simulink model "SE17"  (R2021a)
settings: Solver=FixedStepAuto  StartTime=0.0  StopTime=20  FixedStep=.01  RelTol=1e-3
undefined symbols (not defined in the file or in its folder): Ion, Li, r_c, r_D, u_ce0, u_D0
libraries: Lib_EMTAT x26, pid_lib x5
(part 1 of 2)
settings Model: PacingRate=0.100000  Creator=mebell  LastModifiedBy=mebell
settings SolverCC: AlgebraicLoopSolver=TrustRegion
settings DebuggingCC: SFMachineParentedDataDiag=warning

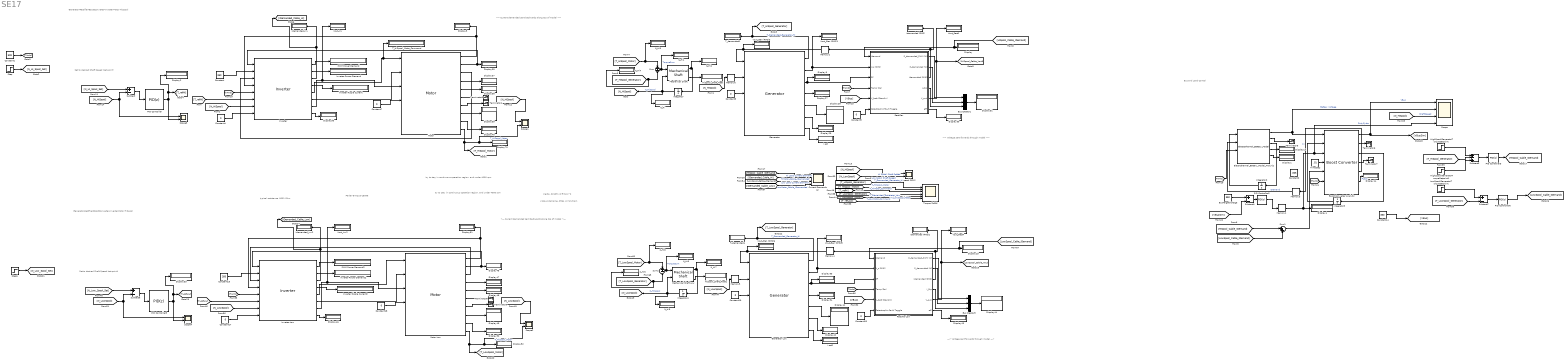
== system SE17 ==
  note: Set to desired Shaft Speed (set point)
  note: Generator-Rectifier-BoostConverter-Inverter-Motor HiSpool
  note: ---> Voltage sent forwards through model --->
  note: <--- Current demanded sent backwards along top of model <---
  note: try to stay in continuous operation region, and under 4000 rpm
  note: Parker GVK210-150N6
  note: typical resistance .0001 Ohm
  note: try to stay in continuous operation region, and under 4000 rpm
  note: viscous damping .2564 x2 Nm/krpm
  note: inertia .02109 x2 ft lbs s^2
  note: Bus and Load Control
  note: Set to desired Shaft Speed (set point)
  note: ---> Voltage sent forwards through model --->
  note: Generator-Rectifier-BoostConverter-Inverter-Motor HiSpool
  note: <--- Current demanded sent backwards along top of model <---
  Boost Converter Analytic : Lib_EMTAT/Components/Physics-Based/Boost Converter  Pdis_M=1  C_M=5e-08  L_M=0.00051  Ron_M=0.784  RC_M=0.26259  RL_M=0.16086  QgTotal_M=4.5e-09  Vdiode_M=0.8  TRise_M=7e-09  TFall_M=2e-09  Fsw_M=250000  Vgate_M=1.7  n_MOSFET=1  MassEst_M=0.37515  TempIn=Celsius  vOut=125  pow=100  minV=47  maxV=53  rippleMode=Use defaults (5% of voltage output and 10% of inductor current)  vRip=.05  iRip=.1  freqMode=Use default frequency (250 kHz)  freq=250e3
      link override DC - DC Converter/Steady State/TemperatureModifiedPerformanceTerm1 /Constant: Value=1
      settings: SourceProductName=EMTAT
  Bus Creator1 : BusCreator  Inputs=3
  Bus Creator3 : BusCreator  Inputs=3
  BusTargetVoltage : Constant  Value=350
  Constant : Constant  Value=350
  Constant1 : Constant  Value=528
  Constant14 : Constant  Value=350
  Constant15 : Constant  Value=350
  Constant{4,7..9,17..20} (8 alike) : Constant  Value=0
  Constant2 : Constant  Value=.005
  Current Demands (A) : Scope  NumInputPorts=4
  Display{,1..2,4..5,9,13..15,27..31,33..53,75} (36 alike) : Display
  Electrothermal_Battery_Model_Analytic : Lib_EMTAT/Components/Physics-Based/Electrothermal_Battery_Model  E0_M=E0_M  Q_M=Q_M  R_M=R_M  K_M=K_M  B_M=B_M  SOC_Init_M=100  A_M=A_M  battery_type_M=Li-Ion  TempIn=Celsius  BWS=on  thermal=on  nameField=Thermal Model
      settings: SourceProductName=EMTAT
  Generator : Lib_EMTAT/Components/Physics-Based/Generator  pp=3  flux_m=0.15995  R_s=0.02  L_s=0.33  P_Fe_Nom=143776.8778  S_nom=4000  T_nom=110  P_out_max=58600  I_max=360.5  P_in_max=81000  T_max=191  MassEst_M=-8670163  Poles_i=6  R_s_i=.02  L_s_i=.330  S_nom_i=4000  T_nom_i=110  P_out_max_i=58600  I_max_i=360.5  P_in_max_i=81000  K_i=50.25  V_nom_i=340  T_max_i=191  CalculatePFe=Compute iron losses automatically  P_Fe_Nom_i=1200  I_nom_i=180  PF_nom_i=0.99  P_Fe_Calc_Flag=1
      settings: SourceProductName=EMTAT
  Generator Low : Lib_EMTAT/Components/Physics-Based/Generator  pp=3  flux_m=0.15995  R_s=0.02  L_s=0.33  P_Fe_Nom=143776.8778  S_nom=4000  T_nom=110  P_out_max=58600  I_max=360.5  P_in_max=81000  T_max=191  MassEst_M=-8670163  Poles_i=6  R_s_i=.02  L_s_i=.330  S_nom_i=4000  T_nom_i=110  P_out_max_i=58600  I_max_i=360.5  P_in_max_i=81000  K_i=50.25  V_nom_i=340  T_max_i=191  CalculatePFe=Compute iron losses automatically  P_Fe_Nom_i=1200  I_nom_i=180  PF_nom_i=0.99  P_Fe_Calc_Flag=1
      settings: SourceProductName=EMTAT
  HiSpool_Shaft_Heat : Display
  HiSpool_Shaft_Heat1 : Display
  HighSpoolGeneratorTorqueSetpoint : Step  Time=7  After=25  SampleTime=0
  HighSpoolGeneratorTorqueSetpoint1 : Step  Time=4  After=-20  SampleTime=0
  I act : Display
  I act2 : Display
  Idemanded (RMS) : Display
  Idemanded (RMS)2 : Display
  Idemanded_inv : Display
  Idemanded_inv2 : Display
  Integrator : Integrator  LimitOutput=on
  Integrator2 : Integrator
  Integrator3 : Integrator
  Integrator4 : Integrator  LimitOutput=on
  "Inverter " : Lib_EMTAT/Components/Physics-Based/Inverter   T_M=[25 175]  u_D_M=[1.16666666666667 0.999999999999998]  u_ce0_M=[0.971428571428571 0.848275862068965]  R_c_M=[0.0285714285714286 0.0551724137931034]  R_D_M=[0.0238095238095238 0.0294117647058824]  E0_M=[6.00000000000002e-05 6.00000000000002e-05]  E1_M=[5.6e-05 5.6e-05]  f_sw_M=20000  L_s_M=0.1  P_max_I=22000  V_phase_I=600  f_sw_I=0  L_s_I=0.1
      settings: SourceProductName=EMTAT
  Inverter Low : Lib_EMTAT/Components/Physics-Based/Inverter   T_M=[25 175]  u_D_M=[1.16666666666667 0.999999999999998]  u_ce0_M=[0.971428571428571 0.848275862068965]  R_c_M=[0.0285714285714286 0.0551724137931034]  R_D_M=[0.0238095238095238 0.0294117647058824]  E0_M=[6.00000000000002e-05 6.00000000000002e-05]  E1_M=[5.6e-05 5.6e-05]  f_sw_M=20000  L_s_M=0.1  P_max_I=22000  V_phase_I=600  f_sw_I=0  L_s_I=0.1
      settings: SourceProductName=EMTAT
  Inverter Power Demand : Display
  Inverter Power Demand2 : Display
  Inverter Ripple Current : Display
  Inverter Ripple Current2 : Display
  LowSpoolGeneratorTorqueSetpoint : Step  Time=12  After=-5  SampleTime=0
  Mechanical Shaft : Lib_EMTAT/Components/Power Flow/Mechanical Shaft  J=.0422  B=.0236
      settings: SourceProductName=EMTAT
      settings: AttributesFormatString=|
      | Mechanical Shaft
      | Version: %<LibraryVersion>
  Mechanical Shaft Low : Lib_EMTAT/Components/Power Flow/Mechanical Shaft  J=.0422  B=.0236
      settings: SourceProductName=EMTAT
      settings: AttributesFormatString=|
      | Mechanical Shaft
      | Version: %<LibraryVersion>
  Memory1 : Memory  InitialCondition=.8
  Memory2 : Memory  InitialCondition=1
  Memory3 : Memory  InitialCondition=.05
  Memory4 : Memory  InitialCondition=1
  Memory5 : Memory  InitialCondition=3000
  Memory6 : Memory  InitialCondition=3000
  "Motor " : Lib_EMTAT/Components/Physics-Based/Motor   pp=6  flux_m=0.079975  R_s=0.02  L_s=0.33  P_Fe_Nom=1200  S_nom=4000  T_nom=110  P_out_max=58600  I_max=360.5  P_in_max=81000  T_max=191  MassEst_M=25  Poles_i=12  R_s_i=.02  L_s_i=.330  S_nom_i=4000  T_nom_i=110  P_out_max_i=58600  I_max_i=360.5  P_in_max_i=81000  K_i=50.25  V_nom_i=340  T_max_i=191  CalculatePFe=Compute iron losses automatically  P_Fe_Nom_i=1200  I_nom_i=180  PF_nom_i=0.99  P_Fe_Calc_Flag=1
      settings: SourceProductName=EMTAT
  Motor Low : Lib_EMTAT/Components/Physics-Based/Motor   pp=6  flux_m=0.079975  R_s=0.02  L_s=0.33  P_Fe_Nom=1200  S_nom=4000  T_nom=110  P_out_max=58600  I_max=360.5  P_in_max=81000  T_max=191  MassEst_M=25  Poles_i=12  R_s_i=.02  L_s_i=.330  S_nom_i=4000  T_nom_i=110  P_out_max_i=58600  I_max_i=360.5  P_in_max_i=81000  K_i=50.25  V_nom_i=340  T_max_i=191  CalculatePFe=Compute iron losses automatically  P_Fe_Nom_i=1200  I_nom_i=180  PF_nom_i=0.99  P_Fe_Calc_Flag=1
      settings: SourceProductName=EMTAT
  N_Hi{,1..9} (10 alike) : Display
  PID Controller : pid_lib/PID Controller  Controller=PID  Form=Parallel  TimeDomain=Discrete-time  UseExternalTs=off  SampleTime=-1  IntegratorMethod=Forward Euler  FilterMethod=Forward Euler  ControllerParametersSource=internal  P=.05  I=.01  D=0  UseFilter=on  N=100  TunerSelectOption=Transfer Function Based (PID Tuner App)  InitialConditionSource=internal  InitialConditionForIntegrator=0  InitialConditionForFilter=0  DifferentiatorICPrevScaledInput=0  ExternalReset=none  TrackingMode=off  Kt=1  LimitOutput=off  SatLimitsSource=internal  UpperSaturationLimit=inf  LowerSaturationLimit=-inf  LinearizeAsGain=on  AntiWindupMode=none  Kb=1  RndMeth=Round  POutMin=[]  POutMax=[]  IOutMin=[]  IOutMax=[]  DOutMin=[]  DOutMax=[]  NOutMin=[]  NOutMax=[]  SumOutMin=[]  SumOutMax=[]  SaturationOutMin=[]  SaturationOutMax=[]  PParamMin=[]  PParamMax=[]  IParamMin=[]  IParamMax=[]  DParamMin=[]  DParamMax=[]  NParamMin=[]  NParamMax=[]  KbParamMin=[]  KbParamMax=[]  KtParamMin=[]  KtParamMax=[]  KbOutMin=[]  KbOutMax=[]  KtOutMin=[]  KtOutMax=[]  IntegratorOutMin=[]  IntegratorOutMax=[]  FilterOutMin=[]  FilterOutMax=[]  SumI1OutMin=[]  SumI1OutMax=[]  SumI2OutMin=[]  SumI2OutMax=[]  SumI3OutMin=[]  SumI3OutMax=[]  SumI4OutMin=[]  SumI4OutMax=[]  SumDOutMin=[]  SumDOutMax=[]  DifferentiatorOutMin=[]  DifferentiatorOutMax=[]  FilterDiffOutCoefMin=[]  FilterDiffOutCoefMax=[]  ReciprocalOutMin=[]  ReciprocalOutMax=[]  SumDenOutMin=[]  SumDenOutMax=[]  SumNumOutMin=[]  SumNumOutMax=[]  DivideOutMin=[]  DivideOutMax=[]  UdiffTsProdOutMin=[]  UdiffTsProdOutMax=[]  NTsProdOutMin=[]  NTsProdOutMax=[]  UintegralTsProdOutMin=[]  UintegralTsProdOutMax=[]  UngainTsProdOutMin=[]  UngainTsProdOutMax=[]  IntegratorContinuousStateAttributes=''  IntegratorStateMustResolveToSignalObject=off  IntegratorRTWStateStorageClass=Auto  FilterContinuousStateAttributes=''  FilterStateMustResolveToSignalObject=off  FilterRTWStateStorageClass=Auto  ParallelPVariant=InternalParameters  IdealPVariant=Disabled  IVariant=InternalParameters  DVariant=InternalParameters  IntegratorVariant=Discrete  SatVariant=Disabled  AWVariant=Passthrough  PCopyVariant=Disabled  TRVariant=Disabled  FdbkBlocksVariant=Forward  IdealPFdbkVariant=Disabled  SatFdbkVariant=Disabled  DerivativeFilterVariant=ForwardEulerFilter  NVariant=InternalParameters  NCopyVariant=Disabled  FilterICVariant=InternalICsFilter  IntegratorICVariant=InternalICs  ExternalResetVariant=Disabled  TRSumVariant=Passthrough  SumFdbkVariant=Disabled  SumVariant=Sum_PID  TsampFilterVariant=InternalTs  TsampNgainVariant=Passthrough  TsampIntegralVariant=Passthrough  ExternalSaturationOutDataTypeStr=Inherit: Same as second input
  PID Controller2 : pid_lib/PID Controller  Controller=PID  Form=Parallel  TimeDomain=Continuous-time  UseExternalTs=off  SampleTime=-1  IntegratorMethod=Forward Euler  FilterMethod=Forward Euler  ControllerParametersSource=internal  P=.0005  I=.005  D=0  UseFilter=on  N=0  TunerSelectOption=Transfer Function Based (PID Tuner App)  InitialConditionSource=internal  InitialConditionForIntegrator=0  InitialConditionForFilter=0  DifferentiatorICPrevScaledInput=0  ExternalReset=none  TrackingMode=off  Kt=1  LimitOutput=on  SatLimitsSource=internal  UpperSaturationLimit=1  LowerSaturationLimit=-inf  LinearizeAsGain=on  AntiWindupMode=none  Kb=1  POutMin=[]  POutMax=[]  IOutMin=[]  IOutMax=[]  DOutMin=[]  DOutMax=[]  NOutMin=[]  NOutMax=[]  SumOutMin=[]  SumOutMax=[]  SaturationOutMin=[]  SaturationOutMax=[]  PParamMin=[]  PParamMax=[]  IParamMin=[]  IParamMax=[]  DParamMin=[]  DParamMax=[]  NParamMin=[]  NParamMax=[]  KbParamMin=[]  KbParamMax=[]  KtParamMin=[]  KtParamMax=[]  KbOutMin=[]  KbOutMax=[]  KtOutMin=[]  KtOutMax=[]  IntegratorOutMin=[]  IntegratorOutMax=[]  FilterOutMin=[]  FilterOutMax=[]  SumI1OutMin=[]  SumI1OutMax=[]  SumI2OutMin=[]  SumI2OutMax=[]  SumI3OutMin=[]  SumI3OutMax=[]  SumI4OutMin=[]  SumI4OutMax=[]  SumDOutMin=[]  SumDOutMax=[]  DifferentiatorOutMin=[]  DifferentiatorOutMax=[]  FilterDiffOutCoefMin=[]  FilterDiffOutCoefMax=[]  ReciprocalOutMin=[]  ReciprocalOutMax=[]  SumDenOutMin=[]  SumDenOutMax=[]  SumNumOutMin=[]  SumNumOutMax=[]  DivideOutMin=[]  DivideOutMax=[]  UdiffTsProdOutMin=[]  UdiffTsProdOutMax=[]  NTsProdOutMin=[]  NTsProdOutMax=[]  UintegralTsProdOutMin=[]  UintegralTsProdOutMax=[]  UngainTsProdOutMin=[]  UngainTsProdOutMax=[]  IntegratorContinuousStateAttributes=''  IntegratorStateMustResolveToSignalObject=off  IntegratorRTWStateStorageClass=Auto  FilterContinuousStateAttributes=''  FilterStateMustResolveToSignalObject=off  FilterRTWStateStorageClass=Auto  ParallelPVariant=InternalParameters  IdealPVariant=Disabled  IVariant=InternalParameters  DVariant=InternalParameters  IntegratorVariant=Continuous  SatVariant=Enabled  AWVariant=Passthrough  PCopyVariant=Disabled  TRVariant=Disabled  FdbkBlocksVariant=Forward  IdealPFdbkVariant=Disabled  SatFdbkVariant=Disabled  DerivativeFilterVariant=ContFilter  NVariant=InternalParameters  NCopyVariant=Disabled  FilterICVariant=InternalICsFilter  IntegratorICVariant=InternalICs  ExternalResetVariant=Disabled  TRSumVariant=Passthrough  SumFdbkVariant=Disabled  SumVariant=Sum_PID  TsampFilterVariant=InternalTs  TsampNgainVariant=Passthrough  TsampIntegralVariant=Passthrough  ExternalSaturationOutDataTypeStr=Inherit: Same as second input
  PID Controller3 : pid_lib/PID Controller  Controller=PID  Form=Parallel  TimeDomain=Continuous-time  UseExternalTs=off  SampleTime=-1  IntegratorMethod=Forward Euler  FilterMethod=Forward Euler  ControllerParametersSource=internal  P=0  I=1.09  D=0  UseFilter=on  N=100  TunerSelectOption=Transfer Function Based (PID Tuner App)  ZeroCross=off  InitialConditionSource=internal  InitialConditionForIntegrator=0  InitialConditionForFilter=0  DifferentiatorICPrevScaledInput=0  ExternalReset=none  TrackingMode=off  Kt=1  LimitOutput=off  SatLimitsSource=internal  UpperSaturationLimit=inf  LowerSaturationLimit=-inf  LinearizeAsGain=on  AntiWindupMode=none  Kb=1  POutMin=[]  POutMax=[]  IOutMin=[]  IOutMax=[]  DOutMin=[]  DOutMax=[]  NOutMin=[]  NOutMax=[]  SumOutMin=[]  SumOutMax=[]  SaturationOutMin=[]  SaturationOutMax=[]  PParamMin=[]  PParamMax=[]  IParamMin=[]  IParamMax=[]  DParamMin=[]  DParamMax=[]  NParamMin=[]  NParamMax=[]  KbParamMin=[]  KbParamMax=[]  KtParamMin=[]  KtParamMax=[]  KbOutMin=[]  KbOutMax=[]  KtOutMin=[]  KtOutMax=[]  IntegratorOutMin=[]  IntegratorOutMax=[]  FilterOutMin=[]  FilterOutMax=[]  SumI1OutMin=[]  SumI1OutMax=[]  SumI2OutMin=[]  SumI2OutMax=[]  SumI3OutMin=[]  SumI3OutMax=[]  SumI4OutMin=[]  SumI4OutMax=[]  SumDOutMin=[]  SumDOutMax=[]  DifferentiatorOutMin=[]  DifferentiatorOutMax=[]  FilterDiffOutCoefMin=[]  FilterDiffOutCoefMax=[]  ReciprocalOutMin=[]  ReciprocalOutMax=[]  SumDenOutMin=[]  SumDenOutMax=[]  SumNumOutMin=[]  SumNumOutMax=[]  DivideOutMin=[]  DivideOutMax=[]  UdiffTsProdOutMin=[]  UdiffTsProdOutMax=[]  NTsProdOutMin=[]  NTsProdOutMax=[]  UintegralTsProdOutMin=[]  UintegralTsProdOutMax=[]  UngainTsProdOutMin=[]  UngainTsProdOutMax=[]  IntegratorContinuousStateAttributes=''  IntegratorStateMustResolveToSignalObject=off  IntegratorRTWStateStorageClass=Auto  FilterContinuousStateAttributes=''  FilterStateMustResolveToSignalObject=off  FilterRTWStateStorageClass=Auto  ParallelPVariant=InternalParameters  IdealPVariant=Disabled  IVariant=InternalParameters  DVariant=InternalParameters  IntegratorVariant=Continuous  SatVariant=Disabled  AWVariant=Passthrough  PCopyVariant=Disabled  TRVariant=Disabled  FdbkBlocksVariant=Forward  IdealPFdbkVariant=Disabled  SatFdbkVariant=Disabled  DerivativeFilterVariant=ContFilter  NVariant=InternalParameters  NCopyVariant=Disabled  FilterICVariant=InternalICsFilter  IntegratorICVariant=InternalICs  ExternalResetVariant=Disabled  TRSumVariant=Passthrough  SumFdbkVariant=Disabled  SumVariant=Sum_PID  TsampFilterVariant=InternalTs  TsampNgainVariant=Passthrough  TsampIntegralVariant=Passthrough  ExternalSaturationOutDataTypeStr=Inherit: Same as second input
  PID Controller5 : pid_lib/PID Controller  Controller=PID  Form=Parallel  TimeDomain=Discrete-time  UseExternalTs=off  SampleTime=-1  IntegratorMethod=Forward Euler  FilterMethod=Forward Euler  ControllerParametersSource=internal  P=.05  I=.01  D=0  UseFilter=on  N=100  TunerSelectOption=Transfer Function Based (PID Tuner App)  InitialConditionSource=internal  InitialConditionForIntegrator=0  InitialConditionForFilter=0  DifferentiatorICPrevScaledInput=0  ExternalReset=none  TrackingMode=off  Kt=1  LimitOutput=off  SatLimitsSource=internal  UpperSaturationLimit=inf  LowerSaturationLimit=-inf  LinearizeAsGain=on  AntiWindupMode=none  Kb=1  RndMeth=Round  POutMin=[]  POutMax=[]  IOutMin=[]  IOutMax=[]  DOutMin=[]  DOutMax=[]  NOutMin=[]  NOutMax=[]  SumOutMin=[]  SumOutMax=[]  SaturationOutMin=[]  SaturationOutMax=[]  PParamMin=[]  PParamMax=[]  IParamMin=[]  IParamMax=[]  DParamMin=[]  DParamMax=[]  NParamMin=[]  NParamMax=[]  KbParamMin=[]  KbParamMax=[]  KtParamMin=[]  KtParamMax=[]  KbOutMin=[]  KbOutMax=[]  KtOutMin=[]  KtOutMax=[]  IntegratorOutMin=[]  IntegratorOutMax=[]  FilterOutMin=[]  FilterOutMax=[]  SumI1OutMin=[]  SumI1OutMax=[]  SumI2OutMin=[]  SumI2OutMax=[]  SumI3OutMin=[]  SumI3OutMax=[]  SumI4OutMin=[]  SumI4OutMax=[]  SumDOutMin=[]  SumDOutMax=[]  DifferentiatorOutMin=[]  DifferentiatorOutMax=[]  FilterDiffOutCoefMin=[]  FilterDiffOutCoefMax=[]  ReciprocalOutMin=[]  ReciprocalOutMax=[]  SumDenOutMin=[]  SumDenOutMax=[]  SumNumOutMin=[]  SumNumOutMax=[]  DivideOutMin=[]  DivideOutMax=[]  UdiffTsProdOutMin=[]  UdiffTsProdOutMax=[]  NTsProdOutMin=[]  NTsProdOutMax=[]  UintegralTsProdOutMin=[]  UintegralTsProdOutMax=[]  UngainTsProdOutMin=[]  UngainTsProdOutMax=[]  IntegratorContinuousStateAttributes=''  IntegratorStateMustResolveToSignalObject=off  IntegratorRTWStateStorageClass=Auto  FilterContinuousStateAttributes=''  FilterStateMustResolveToSignalObject=off  FilterRTWStateStorageClass=Auto  ParallelPVariant=InternalParameters  IdealPVariant=Disabled  IVariant=InternalParameters  DVariant=InternalParameters  IntegratorVariant=Discrete  SatVariant=Disabled  AWVariant=Passthrough  PCopyVariant=Disabled  TRVariant=Disabled  FdbkBlocksVariant=Forward  IdealPFdbkVariant=Disabled  SatFdbkVariant=Disabled  DerivativeFilterVariant=ForwardEulerFilter  NVariant=InternalParameters  NCopyVariant=Disabled  FilterICVariant=InternalICsFilter  IntegratorICVariant=InternalICs  ExternalResetVariant=Disabled  TRSumVariant=Passthrough  SumFdbkVariant=Disabled  SumVariant=Sum_PID  TsampFilterVariant=InternalTs  TsampNgainVariant=Passthrough  TsampIntegralVariant=Passthrough  ExternalSaturationOutDataTypeStr=Inherit: Same as second input
  PID Controller6 : pid_lib/PID Controller  Controller=PID  Form=Parallel  TimeDomain=Continuous-time  UseExternalTs=off  SampleTime=-1  IntegratorMethod=Forward Euler  FilterMethod=Forward Euler  ControllerParametersSource=internal  P=0  I=1.09  D=0  UseFilter=on  N=100  TunerSelectOption=Transfer Function Based (PID Tuner App)  ZeroCross=off  InitialConditionSource=internal  InitialConditionForIntegrator=0  InitialConditionForFilter=0  DifferentiatorICPrevScaledInput=0  ExternalReset=none  TrackingMode=off  Kt=1  LimitOutput=off  SatLimitsSource=internal  UpperSaturationLimit=inf  LowerSaturationLimit=-inf  LinearizeAsGain=on  AntiWindupMode=none  Kb=1  POutMin=[]  POutMax=[]  IOutMin=[]  IOutMax=[]  DOutMin=[]  DOutMax=[]  NOutMin=[]  NOutMax=[]  SumOutMin=[]  SumOutMax=[]  SaturationOutMin=[]  SaturationOutMax=[]  PParamMin=[]  PParamMax=[]  IParamMin=[]  IParamMax=[]  DParamMin=[]  DParamMax=[]  NParamMin=[]  NParamMax=[]  KbParamMin=[]  KbParamMax=[]  KtParamMin=[]  KtParamMax=[]  KbOutMin=[]  KbOutMax=[]  KtOutMin=[]  KtOutMax=[]  IntegratorOutMin=[]  IntegratorOutMax=[]  FilterOutMin=[]  FilterOutMax=[]  SumI1OutMin=[]  SumI1OutMax=[]  SumI2OutMin=[]  SumI2OutMax=[]  SumI3OutMin=[]  SumI3OutMax=[]  SumI4OutMin=[]  SumI4OutMax=[]  SumDOutMin=[]  SumDOutMax=[]  DifferentiatorOutMin=[]  DifferentiatorOutMax=[]  FilterDiffOutCoefMin=[]  FilterDiffOutCoefMax=[]  ReciprocalOutMin=[]  ReciprocalOutMax=[]  SumDenOutMin=[]  SumDenOutMax=[]  SumNumOutMin=[]  SumNumOutMax=[]  DivideOutMin=[]  DivideOutMax=[]  UdiffTsProdOutMin=[]  UdiffTsProdOutMax=[]  NTsProdOutMin=[]  NTsProdOutMax=[]  UintegralTsProdOutMin=[]  UintegralTsProdOutMax=[]  UngainTsProdOutMin=[]  UngainTsProdOutMax=[]  IntegratorContinuousStateAttributes=''  IntegratorStateMustResolveToSignalObject=off  IntegratorRTWStateStorageClass=Auto  FilterContinuousStateAttributes=''  FilterStateMustResolveToSignalObject=off  FilterRTWStateStorageClass=Auto  ParallelPVariant=InternalParameters  IdealPVariant=Disabled  IVariant=InternalParameters  DVariant=InternalParameters  IntegratorVariant=Continuous  SatVariant=Disabled  AWVariant=Passthrough  PCopyVariant=Disabled  TRVariant=Disabled  FdbkBlocksVariant=Forward  IdealPFdbkVariant=Disabled  SatFdbkVariant=Disabled  DerivativeFilterVariant=ContFilter  NVariant=InternalParameters  NCopyVariant=Disabled  FilterICVariant=InternalICsFilter  IntegratorICVariant=InternalICs  ExternalResetVariant=Disabled  TRSumVariant=Passthrough  SumFdbkVariant=Disabled  SumVariant=Sum_PID  TsampFilterVariant=InternalTs  TsampNgainVariant=Passthrough  TsampIntegralVariant=Passthrough  ExternalSaturationOutDataTypeStr=Inherit: Same as second input
  PWM Power Demand : Display
  PWM Power Demand2 : Display
  Rectifier : Subsystem  AncestorBlock=Lib_EMTAT/Components/Physics-Based/Rectifier  mask{T_M=[25 175], u_D_M=[1.16666666666667 0.999999999999998], u_ce0_M=[0.971428571428571 0.848275862068965], R_c_M=[0.0285714285714286 0.0551724137931034], R_D_M=[0.0238095238095238 0.0294117647058824], E0_M=[6.00000000000002e-05 6.00000000000002e-05], E1_M=[5.6e-05 5.6e-05], f_sw_M=20000, L_s_M=0.1, P_max_I=22000, V_phase_I=600, f_sw_I=0, L_s_I=0.1}
      mask prompts: T_M "Temperature Breakpoints (degrees C)"; u_D_M "u_D (Diode voltage at 0A), as a function of T"; u_ce0_M "u_ce0 (IGBT voltage at 0A), as a function of T"; R_c_M "R_c (IGBT resistance), as a function of T"; R_D_M "R_D (Diode resistance), as a linear of T"; E0_M "E0 switching energy coefficient"; E1_M "E1 switching energy coefficient"; f_sw_M "Switching Frequency (Hz)"; L_s_M "Stator Inductance of Attached Motor"; P_max_I "Maximum power"; V_phase_I "Maximum phase voltage (set to 0 to disregard)"; f_sw_I "F_sw (set to 0 to default to maximum for given IGBT)"; L_s_I "Stator inductance of Motor (required for ripple current calculation)"
      mask DialogControl Container4 Prompt: Parameters
      mask DialogControl Control2 Prompt: The way that the above parameters are used is that each vector is 2 long, using points in the linear zone of the curves. Interpolation is used to find values at other temperatures.
      mask DialogControl Container4_copy Prompt: iDesign 1
      mask DialogControl runbutton Prompt: RUN iDESIGN
      mask DialogControl runbutton Callback: run('Run_iDesign_InverterSS')
  Rectifier Low : Subsystem  AncestorBlock=Lib_EMTAT/Components/Physics-Based/Rectifier  mask{T_M=[25 175], u_D_M=[1.16666666666667 0.999999999999998], u_ce0_M=[0.971428571428571 0.848275862068965], R_c_M=[0.0285714285714286 0.0551724137931034], R_D_M=[0.0238095238095238 0.0294117647058824], E0_M=[6.00000000000002e-05 6.00000000000002e-05], E1_M=[5.6e-05 5.6e-05], f_sw_M=20000, L_s_M=0.1, P_max_I=22000, V_phase_I=600, f_sw_I=0, L_s_I=0.1}
      mask prompts: T_M "Temperature Breakpoints (degrees C)"; u_D_M "u_D (Diode voltage at 0A), as a function of T"; u_ce0_M "u_ce0 (IGBT voltage at 0A), as a function of T"; R_c_M "R_c (IGBT resistance), as a function of T"; R_D_M "R_D (Diode resistance), as a linear of T"; E0_M "E0 switching energy coefficient"; E1_M "E1 switching energy coefficient"; f_sw_M "Switching Frequency (Hz)"; L_s_M "Stator Inductance of Attached Motor"; P_max_I "Maximum power"; V_phase_I "Maximum phase voltage (set to 0 to disregard)"; f_sw_I "F_sw (set to 0 to default to maximum for given IGBT)"; L_s_I "Stator inductance of Motor (required for ripple current calculation)"
      mask DialogControl Container4 Prompt: Parameters
      mask DialogControl Control2 Prompt: The way that the above parameters are used is that each vector is 2 long, using points in the linear zone of the curves. Interpolation is used to find values at other temperatures.
      mask DialogControl Container4_copy Prompt: iDesign 1
      mask DialogControl runbutton Prompt: RUN iDESIGN
      mask DialogControl runbutton Callback: run('Run_iDesign_InverterSS')
  Scope : Scope  NumInputPorts=4
  Scope{1..4} (4 alike) : Scope  NumInputPorts=2
  Speed (RPM) : Scope  NumInputPorts=2
  Step : Step  Time=.5  After=4000  SampleTime=0
  Step6 : Step  Time=.75  After=4000  SampleTime=0
  Subtract{,1,6..7} (4 alike) : Sum  Inputs=+-
  Subtract3 : Sum  Inputs=+-+
  Sum : Sum  Inputs=+|-
  Sum1 : Sum  Inputs=|++
  Sum2 : Sum  Inputs=+|-
  T_HiSpool_Motor_Command : Display
  T_demanded1 : Display
  T_demanded4 : Display
  Terminator{3..9} (7 alike) : Terminator
  TimeStep : Constant  Value=.01
  Torque (lbf-ft) : Scope  NumInputPorts=6
  Vout_Gen (RMS){1,3,5..6} (4 alike) : Display
  Vout_Inv : Display
  Vout_Inv2 : Display
  Vout_Rect1 : Display
  Vout_Rect4 : Display
  wires:
  "Inverter "/6 -> "Motor "/2
  Generator/4 -> Display27/1
  "Motor "/3 -> "Inverter "/3
  Constant1/1 -> [TAmb]
  "Inverter "/7 -> "Motor "/3, Vout_Inv/1
  "Motor "/2 -> "Inverter "/1, Display35/1
  "Motor "/10 -> Scope1/2, Display75/1, [T_HiSpool_Motor]  "T_HiSpool_Motor"
  "Motor "/8 -> Display39/1
  Rectifier/1(P_demanded_PWM (W)) -> Bus Creator1/1
  Generator/7 -> I act/1
  [T_refHi] -> "Inverter "/6
  [TAmb] -> "Inverter "/5
  Rectifier/4(I_Rip) -> Bus Creator1/3
  Bus Creator1/1 -> Display31/1
  Generator/5 -> Display28/1
  Rectifier/5(V_out) -> [HiSpool_Cable_Vout], Vout_Rect1/1
  Generator/3 -> Rectifier/3(PF), Display9/1
  [TAmb] -> Rectifier/4(Temp (Ra))
  Rectifier/6(eff) -> Display30/1
  "Motor "/5 -> Display38/1
  "Motor "/4 -> Display37/1
  "Motor "/9 -> Display40/1
  Generator/6 -> Display29/1
  [N_HiSpool] -> "Inverter "/7
  [N_HiSpool] -> Memory6/1
  "Inverter "/3 -> [IDemanded_Cable_Hi], Idemanded_inv/1
  "Inverter "/8 -> Display36/1
  Rectifier/2(P_demanded (W)) -> Bus Creator1/2
  Rectifier/3(Idemanded (RMS)) -> Idemanded (RMS)/1, Memory2/1
  "Inverter "/5 -> T_HiSpool_Motor_Command/1, "Motor "/1
  Generator/1 -> [T_HiSpool_Generator], T_demanded1/1  "T_Demanded_Generator_Hi"
  Sum/1 -> N_Hi1/1, Mechanical Shaft/1  "TorqueSum"
  Constant/1 -> "Inverter "/2
  [T_HiSpool_Motor] -> N_Hi3/1, Sum/1
  [T_HiSpool_Generator] -> N_Hi4/1, Sum/2
  Mechanical Shaft/3 -> HiSpool_Shaft_Heat/1
  [N_Hi_Spool_Set] -> Subtract/1
  [HiSpool_Cable_IDemand] -> Rectifier/1(Idemand), Display/1
  "Motor "/1 -> "Inverter "/4, Display5/1
  Mechanical Shaft/1 -> N_Hi2/1, Integrator/1
  Integrator/1 -> N_Hi/1, Mechanical Shaft/2, [N_HiSpool]  "N_HiSpool"
  [N_HiSpool] -> Scope1/1
  Generator/2 -> Rectifier/2("V_s (RMS) "), Vout_Gen (RMS)1/1
  [N_HiSpool] -> Speed (RPM)/1  "Hi Spool Shaft Speed"
  PID Controller/1 -> Scope3/2, Display2/1, [T_refHi]
  [N_HiSpool] -> Scope3/1, Subtract/2
  Subtract/1 -> PID Controller/1
  "Inverter "/1 -> PWM Power Demand/1
  "Inverter "/2 -> Inverter Power Demand/1
  Memory6/1 -> Generator/2
  [T_refHi] -> Torque (lbf-ft)/3  "T_HiMotor_Command"
  [HiSpool_Cable_IDemand] -> Current Demands (A)/1  "Hi Load Current Demand"
  [T_HiSpool_Generator] -> Torque (lbf-ft)/1  "T_Demanded_Generator_Hi"
  "Inverter "/4 -> Inverter Ripple Current/1
  "Motor "/7 -> Terminator4/1
  "Motor "/6 -> Terminator3/1
  [TAmb] -> Electrothermal_Battery_Model_Analytic/3
  Electrothermal_Battery_Model_Analytic/1 -> Boost Converter Analytic/1, Scope/2  "Battery Voltage"
  Electrothermal_Battery_Model_Analytic/3 -> Integrator2/1
  Integrator2/1 -> Electrothermal_Battery_Model_Analytic/1
  Electrothermal_Battery_Model_Analytic/2 -> Terminator5/1
  Boost Converter Analytic/5 -> Memory3/1  "Iin"
  Boost Converter Analytic/6 -> Display14/1  "PLoss"
  Electrothermal_Battery_Model_Analytic/4 -> Display13/1
  Boost Converter Analytic/3 -> Integrator3/1
  Integrator3/1 -> Boost Converter Analytic/2
  Boost Converter Analytic/2 -> Terminator6/1
  Boost Converter Analytic/1 -> [VBusSim], Scope/1  "VBus"
  [VBus] -> Rectifier/5(V_batt (Standin))
  Subtract1/1 -> PID Controller2/1
  BusTargetVoltage/1 -> Subtract1/1
  [VBusSim] -> Subtract1/2
  PID Controller2/1 -> Memory1/1
  TimeStep/1 -> Boost Converter Analytic/4
  [TAmb] -> Boost Converter Analytic/6
  Boost Converter Analytic/4 -> Terminator7/1
  Sum1/1 -> Boost Converter Analytic/5
  [N_HiSpool] -> Scope/3  "ShaftSpeed"
  Memory3/1 -> Electrothermal_Battery_Model_Analytic/2  "IDemand"
  Memory1/1 -> Display4/1, Scope/4, Boost Converter Analytic/3  "DutyCycle"
  Step/1 -> [N_Hi_Spool_Set]
  [IDemanded_Cable_Hi] -> Current Demands (A)/2  "HiMotor_Cable_IDemanded"
  Constant4/1 -> "Inverter "/8
  Constant7/1 -> "Motor "/4
  Constant8/1 -> Generator/3
  Constant9/1 -> Rectifier/6(Catastrophic Fault Toggle)
  Memory2/1 -> Vout_Gen (RMS)3/1, Generator/1
  PID Controller3/1 -> [HiSpool_Cable_IDemand]
  Subtract3/1 -> PID Controller3/1
  [T_HiSpool_Generator] -> Subtract3/2
  HighSpoolGeneratorTorqueSetpoint/1 -> Subtract3/1
  Constant14/1 -> [VBus]
  [T_LowSpool_Motor] -> Torque (lbf-ft)/5  "T_LowSpool_Motor"
  [T_HiSpool_Motor] -> Torque (lbf-ft)/2  "T_HiSpool_Motor"
  Mechanical Shaft Low/1 -> N_Hi7/1, Integrator4/1
  Motor Low/5 -> Display48/1
  [LowSpool_Cable_IDemand] -> Rectifier Low/1(Idemand), Display15/1
  Rectifier Low/1(P_demanded_PWM (W)) -> Bus Creator3/1
  Rectifier Low/2(P_demanded (W)) -> Bus Creator3/2
  [TAmb] -> Rectifier Low/4(Temp (Ra))
  Memory4/1 -> Vout_Gen (RMS)6/1, Generator Low/1
  Mechanical Shaft Low/3 -> HiSpool_Shaft_Heat1/1
  Generator Low/2 -> Rectifier Low/2("V_s (RMS) "), Vout_Gen (RMS)5/1
  [N_LowSpool] -> Scope2/1
  Motor Low/1 -> Inverter Low/4, Display51/1
  [N_LowSpool] -> Speed (RPM)/2  "Low Spool Shaft Speed"
  [LowSpool_Cable_IDemand] -> Current Demands (A)/3  "Low Load Current Demand"
  Inverter Low/2 -> Inverter Power Demand2/1
  Generator Low/7 -> I act2/1
  Memory5/1 -> Generator Low/2
  Rectifier Low/3(Idemanded (RMS)) -> Idemanded (RMS)2/1, Memory4/1
  [N_Low_Spool_Set] -> Subtract6/1
  Constant15/1 -> Inverter Low/2
  Inverter Low/1 -> PWM Power Demand2/1
  Subtract6/1 -> PID Controller5/1
  [T_LowSpool_Generator] -> N_Hi9/1, Sum2/2
  Generator Low/1 -> [T_LowSpool_Generator], T_demanded4/1  "T_Demanded_Generator_Hi"
  Inverter Low/3 -> [IDemanded_Cable_Low], Idemanded_inv2/1
  Inverter Low/8 -> Display46/1
  [N_LowSpool] -> Memory5/1
  Generator Low/5 -> Display41/1
  Motor Low/10 -> Scope2/2, Display52/1, [T_LowSpool_Motor]  "T_HiSpool_Motor"
  Motor Low/8 -> Display49/1
  Generator Low/4 -> Display34/1
  Integrator4/1 -> N_Hi5/1, Mechanical Shaft Low/2, [N_LowSpool]  "N_HiSpool"
  Generator Low/3 -> Rectifier Low/3(PF), Display53/1
  Motor Low/9 -> Display50/1
  Constant18/1 -> Motor Low/4
  Constant17/1 -> Inverter Low/8
  [IDemanded_Cable_Low] -> Current Demands (A)/4  "LowMotor_Cable_IDemanded"
  Bus Creator3/1 -> Display44/1
  [T_LowSpool_Generator] -> Torque (lbf-ft)/4  "T_Demanded_Generator_Low"
  [N_LowSpool] -> Scope4/1, Subtract6/2
  Constant20/1 -> Rectifier Low/6(Catastrophic Fault Toggle)
  Step6/1 -> [N_Low_Spool_Set]
  [T_refLow] -> Inverter Low/6
  Rectifier Low/6(eff) -> Display43/1
  Constant19/1 -> Generator Low/3
  PID Controller5/1 -> Scope4/2, Display33/1, [T_refLow]
  Motor Low/3 -> Inverter Low/3
  [VBus] -> Rectifier Low/5(V_batt (Standin))
  Rectifier Low/4(I_Rip) -> Bus Creator3/3
  Inverter Low/7 -> Motor Low/3, Vout_Inv2/1
  Inverter Low/4 -> Inverter Ripple Current2/1
  [N_LowSpool] -> Inverter Low/7
  [T_LowSpool_Motor] -> N_Hi8/1, Sum2/1
  Motor Low/6 -> Terminator8/1
  Inverter Low/5 -> Motor Low/1
  Motor Low/2 -> Inverter Low/1, Display45/1
  Rectifier Low/5(V_out) -> [LowSpool_Cable_Vout], Vout_Rect4/1
  Motor Low/7 -> Terminator9/1
  Generator Low/6 -> Display42/1
  Motor Low/4 -> Display47/1
  [T_refLow] -> Torque (lbf-ft)/6  "T_LowMotor_Command"
  [TAmb] -> Inverter Low/5
  Inverter Low/6 -> Motor Low/2
  Sum2/1 -> N_Hi6/1, Mechanical Shaft Low/1  "TorqueSum"
  [T_LowSpool_Generator] -> Subtract7/2
  PID Controller6/1 -> [LowSpool_Cable_IDemand]
  Subtract7/1 -> PID Controller6/1
  LowSpoolGeneratorTorqueSetpoint/1 -> Subtract7/1
  HighSpoolGeneratorTorqueSetpoint1/1 -> Subtract3/3
  [HiSpool_Cable_IDemand] -> Sum1/1
  [LowSpool_Cable_IDemand] -> Sum1/2
  Electrothermal_Battery_Model_Analytic/5 -> Display1/1

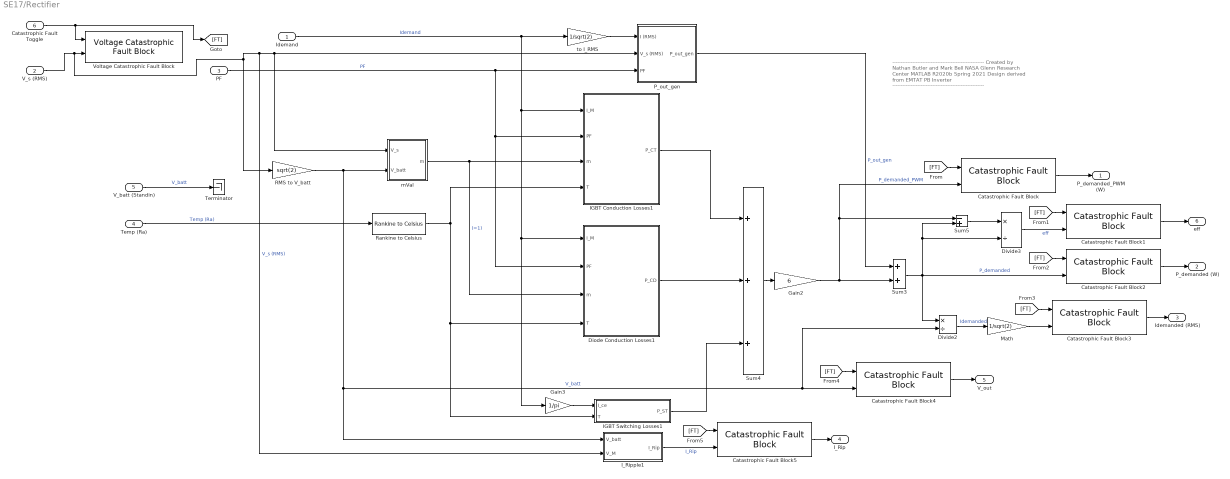
== system SE17/Rectifier ==
  note: -------------------------------------------------------
      | Created by Nathan Butler and Mark Bell
      | NASA Glenn Research Center
      | MATLAB R2020b
      | Spring 2021
      |
      | Design derived from EMTAT PB Inverter
      | -------------------------------------------------------
  Idemand : Inport
  "V_s (RMS) " : Inport  Port=2
  PF : Inport  Port=3
  Temp (Ra) : Inport  Port=4
  V_batt (Standin) : Inport  Port=5
  Catastrophic Fault Toggle : Inport  Port=6
  Catastrophic Fault Block{,1..5} (6 alike) : Lib_EMTAT/Components/Physics-Based/Catastrophic Fault Block  SystemSampleTime=-1  VariantActivationTime=update diagram  Latency=0  AutoFrameSizeCalculation=off
      settings: SourceProductName=EMTAT
  Diode Conduction Losses1 : Subsystem
  Divide2 : Product  Inputs=*/
  Divide3 : Product  Inputs=*/
  Gain2 : Gain  Gain=6
  Gain3 : Gain  Gain=1/pi
  IGBT Conduction Losses1 : Subsystem
  IGBT Switching Losses1 : Subsystem
  I_Ripple1 : Subsystem
  Math : Gain  Gain=1/sqrt(2)
  P_out_gen : Subsystem
  "RMS to V_batt " : Gain  Gain=sqrt(2)
  Rankine to Celsius : Lib_EMTAT/Components/Physics-Based/Rankine to Celsius  SystemSampleTime=-1  VariantActivationTime=update diagram  Latency=0  AutoFrameSizeCalculation=off
      settings: SourceProductName=EMTAT
  Sum3 : Sum
  Sum4 : Sum  Inputs=+++
  Sum5 : Sum  Inputs=-+
  Terminator : Terminator
  Voltage Catastrophic Fault Block : Lib_EMTAT/Components/Physics-Based/Voltage Catastrophic Fault Block  SystemSampleTime=-1  VariantActivationTime=update diagram  Latency=0  AutoFrameSizeCalculation=off
      settings: SourceProductName=EMTAT
  mVal : Subsystem
  to I_RMS : Gain  Gain=1/sqrt(2)
  P_demanded_PWM (W) : Outport  VectorParamsAs1DForOutWhenUnconnected=off
  P_demanded (W) : Outport  Port=2  VectorParamsAs1DForOutWhenUnconnected=off
  Idemanded (RMS) : Outport  Port=3  VectorParamsAs1DForOutWhenUnconnected=off
  I_Rip : Outport  Port=4  VectorParamsAs1DForOutWhenUnconnected=off
  V_out : Outport  Port=5  VectorParamsAs1DForOutWhenUnconnected=off
  eff : Outport  Port=6  VectorParamsAs1DForOutWhenUnconnected=off
  wires:
  "V_s (RMS) "/1 -> P_out_gen/2(V_s (RMS)), mVal/1(V_s), I_Ripple1/2("V_M "), "RMS to V_batt "/1, Voltage Catastrophic Fault Block/2  "V_s (RMS)"
  Catastrophic Fault Toggle/1 -> [FT], Voltage Catastrophic Fault Block/1
  Catastrophic Fault Block5/1 -> I_Rip/1
  I_Ripple1/1(I_Rip) -> Catastrophic Fault Block5/2  "I_Rip"
  [FT] -> Catastrophic Fault Block5/1
  Catastrophic Fault Block4/1 -> V_out/1
  [FT] -> Catastrophic Fault Block4/1
  Catastrophic Fault Block3/1 -> Idemanded (RMS)/1
  Math/1 -> Catastrophic Fault Block3/2
  [FT] -> Catastrophic Fault Block3/1
  Catastrophic Fault Block2/1 -> P_demanded (W)/1
  [FT] -> Catastrophic Fault Block2/1
  Catastrophic Fault Block1/1 -> eff/1
  Divide3/1 -> Catastrophic Fault Block1/2  "eff"
  [FT] -> Catastrophic Fault Block1/1
  [FT] -> Catastrophic Fault Block/1
  Catastrophic Fault Block/1 -> P_demanded_PWM (W)/1
  V_batt (Standin)/1 -> Terminator/1  "V_batt"
  to I_RMS/1 -> P_out_gen/1(I (RMS))
  Sum5/1 -> Divide3/1
  Sum3/1 -> Divide2/1, Sum5/2, Divide3/2, Catastrophic Fault Block2/2  "P_demanded"
  Temp (Ra)/1 -> Rankine to Celsius/1  "Temp (Ra)"
  Gain3/1 -> IGBT Switching Losses1/1(I_ce)
  IGBT Switching Losses1/1(P_ST) -> Sum4/3
  IGBT Conduction Losses1/1(P_CT) -> Sum4/1
  Sum4/1 -> Gain2/1
  Diode Conduction Losses1/1(P_CD) -> Sum4/2
  mVal/1(m) -> IGBT Conduction Losses1/3(m), Diode Conduction Losses1/3(m)  "(=1)"
  PF/1 -> IGBT Conduction Losses1/2(PF), Diode Conduction Losses1/2(PF), P_out_gen/3(PF)  "PF"
  Idemand/1 -> to I_RMS/1, Diode Conduction Losses1/1(I_M), Gain3/1, IGBT Conduction Losses1/1(I_M)  "Idemand"
  Gain2/1 -> Sum5/1, Catastrophic Fault Block/2, Sum3/2  "P_demanded_PWM"
  P_out_gen/1(P_out_gen) -> Sum3/1  "P_out_gen"
  Divide2/1 -> Math/1  "Idemanded"
  "RMS to V_batt "/1 -> mVal/2(V_batt), I_Ripple1/1(V_batt), Divide2/2, Catastrophic Fault Block4/2  "V_batt"
  Rankine to Celsius/1 -> Diode Conduction Losses1/4(T), IGBT Switching Losses1/2(T), IGBT Conduction Losses1/4(T)

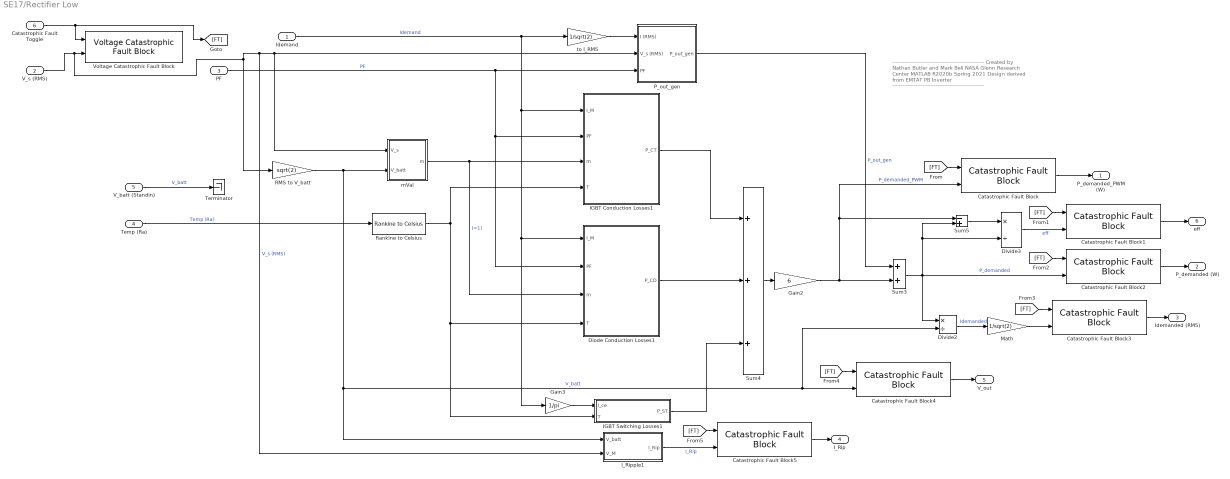
== system SE17/Rectifier Low ==
  note: -------------------------------------------------------
      | Created by Nathan Butler and Mark Bell
      | NASA Glenn Research Center
      | MATLAB R2020b
      | Spring 2021
      |
      | Design derived from EMTAT PB Inverter
      | -------------------------------------------------------
  Idemand : Inport
  "V_s (RMS) " : Inport  Port=2
  PF : Inport  Port=3
  Temp (Ra) : Inport  Port=4
  V_batt (Standin) : Inport  Port=5
  Catastrophic Fault Toggle : Inport  Port=6
  Catastrophic Fault Block{,1..5} (6 alike) : Lib_EMTAT/Components/Physics-Based/Catastrophic Fault Block  SystemSampleTime=-1  VariantActivationTime=update diagram  Latency=0  AutoFrameSizeCalculation=off
      settings: SourceProductName=EMTAT
  Diode Conduction Losses1 : Subsystem
  Divide2 : Product  Inputs=*/
  Divide3 : Product  Inputs=*/
  Gain2 : Gain  Gain=6
  Gain3 : Gain  Gain=1/pi
  IGBT Conduction Losses1 : Subsystem
  IGBT Switching Losses1 : Subsystem
  I_Ripple1 : Subsystem
  Math : Gain  Gain=1/sqrt(2)
  P_out_gen : Subsystem
  "RMS to V_batt " : Gain  Gain=sqrt(2)
  Rankine to Celsius : Lib_EMTAT/Components/Physics-Based/Rankine to Celsius  SystemSampleTime=-1  VariantActivationTime=update diagram  Latency=0  AutoFrameSizeCalculation=off
      settings: SourceProductName=EMTAT
  Sum3 : Sum
  Sum4 : Sum  Inputs=+++
  Sum5 : Sum  Inputs=-+
  Terminator : Terminator
  Voltage Catastrophic Fault Block : Lib_EMTAT/Components/Physics-Based/Voltage Catastrophic Fault Block  SystemSampleTime=-1  VariantActivationTime=update diagram  Latency=0  AutoFrameSizeCalculation=off
      settings: SourceProductName=EMTAT
  mVal : Subsystem
  to I_RMS : Gain  Gain=1/sqrt(2)
  P_demanded_PWM (W) : Outport  VectorParamsAs1DForOutWhenUnconnected=off
  P_demanded (W) : Outport  Port=2  VectorParamsAs1DForOutWhenUnconnected=off
  Idemanded (RMS) : Outport  Port=3  VectorParamsAs1DForOutWhenUnconnected=off
  I_Rip : Outport  Port=4  VectorParamsAs1DForOutWhenUnconnected=off
  V_out : Outport  Port=5  VectorParamsAs1DForOutWhenUnconnected=off
  eff : Outport  Port=6  VectorParamsAs1DForOutWhenUnconnected=off
  wires:
  "V_s (RMS) "/1 -> P_out_gen/2(V_s (RMS)), mVal/1(V_s), I_Ripple1/2("V_M "), "RMS to V_batt "/1, Voltage Catastrophic Fault Block/2  "V_s (RMS)"
  Catastrophic Fault Toggle/1 -> [FT], Voltage Catastrophic Fault Block/1
  Catastrophic Fault Block5/1 -> I_Rip/1
  I_Ripple1/1(I_Rip) -> Catastrophic Fault Block5/2  "I_Rip"
  [FT] -> Catastrophic Fault Block5/1
  Catastrophic Fault Block4/1 -> V_out/1
  [FT] -> Catastrophic Fault Block4/1
  Catastrophic Fault Block3/1 -> Idemanded (RMS)/1
  Math/1 -> Catastrophic Fault Block3/2
  [FT] -> Catastrophic Fault Block3/1
  Catastrophic Fault Block2/1 -> P_demanded (W)/1
  [FT] -> Catastrophic Fault Block2/1
  Catastrophic Fault Block1/1 -> eff/1
  Divide3/1 -> Catastrophic Fault Block1/2  "eff"
  [FT] -> Catastrophic Fault Block1/1
  [FT] -> Catastrophic Fault Block/1
  Catastrophic Fault Block/1 -> P_demanded_PWM (W)/1
  V_batt (Standin)/1 -> Terminator/1  "V_batt"
  to I_RMS/1 -> P_out_gen/1(I (RMS))
  Sum5/1 -> Divide3/1
  Sum3/1 -> Divide2/1, Sum5/2, Divide3/2, Catastrophic Fault Block2/2  "P_demanded"
  Temp (Ra)/1 -> Rankine to Celsius/1  "Temp (Ra)"
  Gain3/1 -> IGBT Switching Losses1/1(I_ce)
  IGBT Switching Losses1/1(P_ST) -> Sum4/3
  IGBT Conduction Losses1/1(P_CT) -> Sum4/1
  Sum4/1 -> Gain2/1
  Diode Conduction Losses1/1(P_CD) -> Sum4/2
  mVal/1(m) -> IGBT Conduction Losses1/3(m), Diode Conduction Losses1/3(m)  "(=1)"
  PF/1 -> IGBT Conduction Losses1/2(PF), Diode Conduction Losses1/2(PF), P_out_gen/3(PF)  "PF"
  Idemand/1 -> to I_RMS/1, Diode Conduction Losses1/1(I_M), Gain3/1, IGBT Conduction Losses1/1(I_M)  "Idemand"
  Gain2/1 -> Sum5/1, Catastrophic Fault Block/2, Sum3/2  "P_demanded_PWM"
  P_out_gen/1(P_out_gen) -> Sum3/1  "P_out_gen"
  Divide2/1 -> Math/1  "Idemanded"
  "RMS to V_batt "/1 -> mVal/2(V_batt), I_Ripple1/1(V_batt), Divide2/2, Catastrophic Fault Block4/2  "V_batt"
  Rankine to Celsius/1 -> Diode Conduction Losses1/4(T), IGBT Switching Losses1/2(T), IGBT Conduction Losses1/4(T)

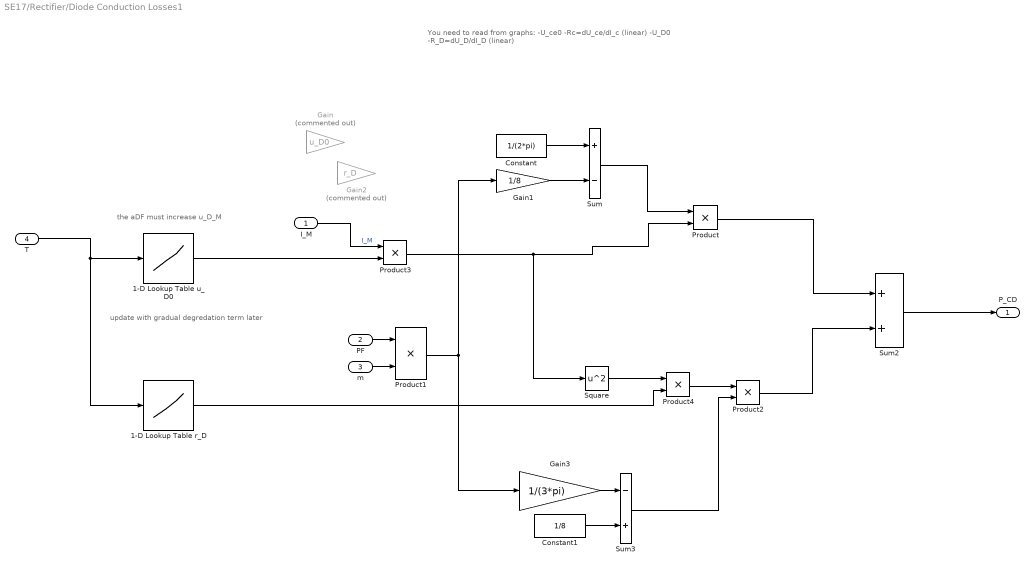
== system SE17/Rectifier/Diode Conduction Losses1 ==
  note: You need to read from graphs:
      |
      | -U_ce0
      | -Rc=dU_ce/dI_c (linear)
      | -U_D0
      | -R_D=dU_D/dI_D (linear)
  note: the aDF must increase u_D_M
  note: update with gradual degredation term later
  I_M : Inport
  PF : Inport  Port=2
  m : Inport  Port=3
  T : Inport  Port=4
  1-D Lookup Table r_D : Lookup_n-D  NumberOfTableDimensions=1  BreakpointsForDimension1=T_M  Table=R_D_M  InternalRulePriority=Speed  RndMeth=Simplest  InputSameDT=on
  1-D Lookup Table u_D0 : Lookup_n-D  NumberOfTableDimensions=1  BreakpointsForDimension1=T_M  Table=u_D_M  InternalRulePriority=Speed  RndMeth=Simplest  InputSameDT=on
  Constant : Constant  Value=1/(2*pi)
  Constant1 : Constant  Value=1/8
  Gain : Gain  Commented=on  Gain=u_D0
  Gain1 : Gain  Gain=1/8
  Gain2 : Gain  Commented=on  Gain=r_D
  Gain3 : Gain  Gain=1/(3*pi)
  Product{,1..4} (5 alike) : Product
  Square : Math  Operator=square  SignedPower=on  SaturateOnIntegerOverflow=on
  Sum : Sum  Inputs=+-
  Sum2 : Sum
  Sum3 : Sum  Inputs=-+
  P_CD : Outport  VectorParamsAs1DForOutWhenUnconnected=off
  wires:
  Product/1 -> Sum2/1
  Product2/1 -> Sum2/2
  Sum2/1 -> P_CD/1
  I_M/1 -> Product3/1  "I_M"
  Product3/1 -> Product/2, Square/1
  Constant/1 -> Sum/1
  PF/1 -> Product1/1
  m/1 -> Product1/2
  Gain1/1 -> Sum/2
  Product1/1 -> Gain3/1, Gain1/1
  Sum/1 -> Product/1
  Square/1 -> Product4/1
  Gain3/1 -> Sum3/1
  Product4/1 -> Product2/1
  Constant1/1 -> Sum3/2
  Sum3/1 -> Product2/2
  T/1 -> 1-D Lookup Table u_D0/1, 1-D Lookup Table r_D/1
  1-D Lookup Table u_D0/1 -> Product3/2
  1-D Lookup Table r_D/1 -> Product4/2

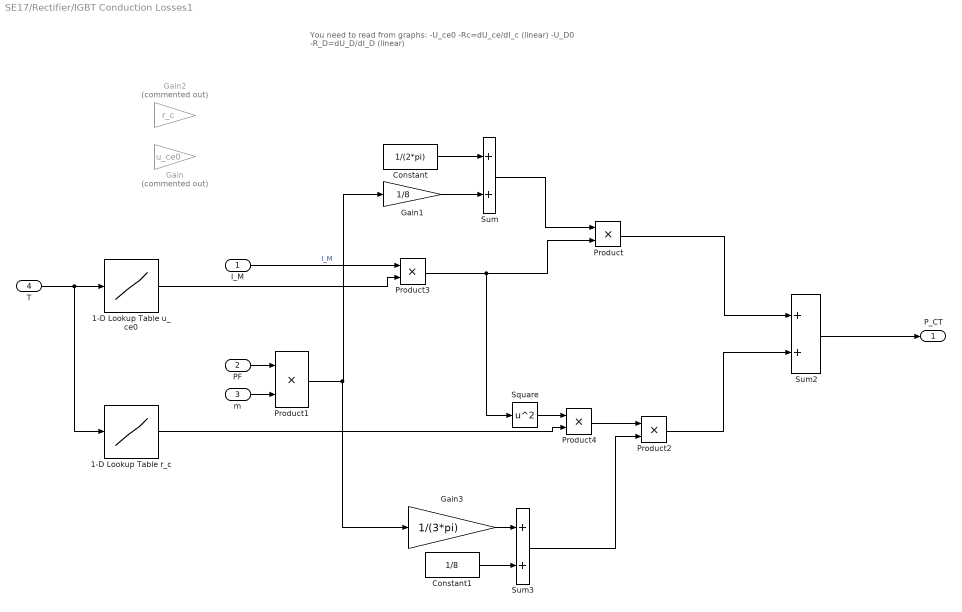
== system SE17/Rectifier/IGBT Conduction Losses1 ==
  note: You need to read from graphs:
      |
      | -U_ce0
      | -Rc=dU_ce/dI_c (linear)
      | -U_D0
      | -R_D=dU_D/dI_D (linear)
  I_M : Inport
  PF : Inport  Port=2
  m : Inport  Port=3
  T : Inport  Port=4
  1-D Lookup Table r_c : Lookup_n-D  NumberOfTableDimensions=1  BreakpointsForDimension1=T_M  Table=R_c_M  InternalRulePriority=Speed  RndMeth=Simplest  InputSameDT=on
  1-D Lookup Table u_ce0 : Lookup_n-D  NumberOfTableDimensions=1  BreakpointsForDimension1=T_M  Table=u_ce0_M  InternalRulePriority=Speed  RndMeth=Simplest  InputSameDT=on
  Constant : Constant  Value=1/(2*pi)
  Constant1 : Constant  Value=1/8
  Gain : Gain  Commented=on  Gain=u_ce0
  Gain1 : Gain  Gain=1/8
  Gain2 : Gain  Commented=on  Gain=r_c
  Gain3 : Gain  Gain=1/(3*pi)
  Product{,1..4} (5 alike) : Product
  Square : Math  Operator=square  SignedPower=on  SaturateOnIntegerOverflow=on
  Sum : Sum
  Sum2 : Sum
  Sum3 : Sum
  P_CT : Outport  VectorParamsAs1DForOutWhenUnconnected=off
  wires:
  Product/1 -> Sum2/1
  Product2/1 -> Sum2/2
  Sum2/1 -> P_CT/1
  I_M/1 -> Product3/1  "I_M"
  Product3/1 -> Product/2, Square/1
  Constant/1 -> Sum/1
  PF/1 -> Product1/1
  m/1 -> Product1/2
  Gain1/1 -> Sum/2
  Product1/1 -> Gain3/1, Gain1/1
  Sum/1 -> Product/1
  Square/1 -> Product4/1
  Gain3/1 -> Sum3/1
  Product4/1 -> Product2/1
  Constant1/1 -> Sum3/2
  Sum3/1 -> Product2/2
  T/1 -> 1-D Lookup Table u_ce0/1, 1-D Lookup Table r_c/1
  1-D Lookup Table u_ce0/1 -> Product3/2
  1-D Lookup Table r_c/1 -> Product4/2

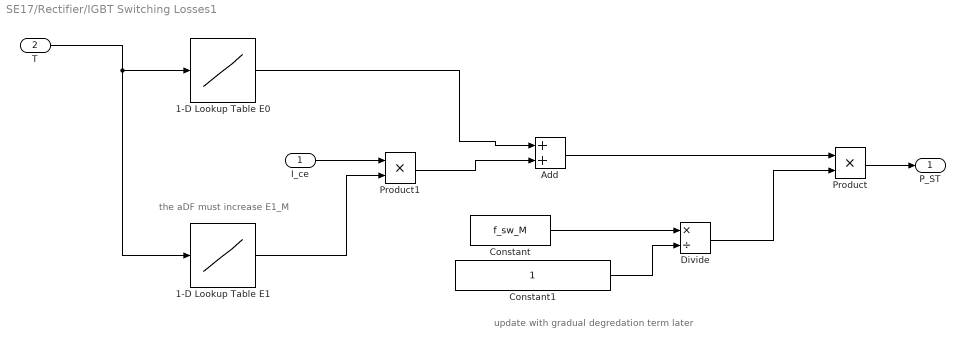
== system SE17/Rectifier/IGBT Switching Losses1 ==
  note: update with gradual degredation term later
  note: the aDF must increase E1_M
  I_ce : Inport
  T : Inport  Port=2
  1-D Lookup Table E0 : Lookup_n-D  NumberOfTableDimensions=1  BreakpointsForDimension1=T_M  Table=E0_M  InternalRulePriority=Speed  RndMeth=Simplest  InputSameDT=on
  1-D Lookup Table E1 : Lookup_n-D  NumberOfTableDimensions=1  BreakpointsForDimension1=T_M  Table=E1_M  InternalRulePriority=Speed  RndMeth=Simplest  InputSameDT=on
  Add : Sum
  Constant : Constant  Value=f_sw_M
  Constant1 : Constant
  Divide : Product  Inputs=*/
  Product : Product
  Product1 : Product
  P_ST : Outport  VectorParamsAs1DForOutWhenUnconnected=off
  wires:
  Constant1/1 -> Divide/2
  Divide/1 -> Product/2
  Constant/1 -> Divide/1
  1-D Lookup Table E1/1 -> Product1/2
  T/1 -> 1-D Lookup Table E1/1, 1-D Lookup Table E0/1
  Product1/1 -> Add/2
  1-D Lookup Table E0/1 -> Add/1
  I_ce/1 -> Product1/1
  Add/1 -> Product/1
  Product/1 -> P_ST/1

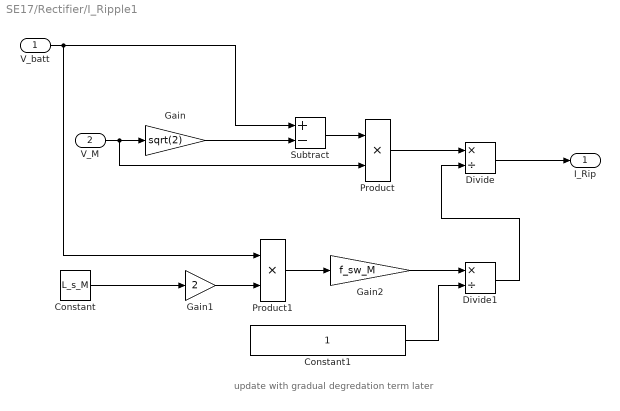
== system SE17/Rectifier/I_Ripple1 ==
  note: update with gradual degredation term later
  V_batt : Inport
  "V_M " : Inport  Port=2
  Constant : Constant  Value=L_s_M
  Constant1 : Constant
  Divide : Product  Inputs=*/
  Divide1 : Product  Inputs=*/
  Gain : Gain  Gain=sqrt(2)
  Gain1 : Gain  Gain=2
  Gain2 : Gain  Gain=f_sw_M
  Product : Product
  Product1 : Product
  Subtract : Sum  Inputs=+-
  I_Rip : Outport  VectorParamsAs1DForOutWhenUnconnected=off
  wires:
  Divide1/1 -> Divide/2
  Constant1/1 -> Divide1/2
  Gain2/1 -> Divide1/1
  "V_M "/1 -> Product/2, Gain/1
  Gain/1 -> Subtract/2
  V_batt/1 -> Subtract/1, Product1/1
  Subtract/1 -> Product/1
  Product/1 -> Divide/1
  Constant/1 -> Gain1/1
  Gain1/1 -> Product1/2
  Product1/1 -> Gain2/1
  Divide/1 -> I_Rip/1

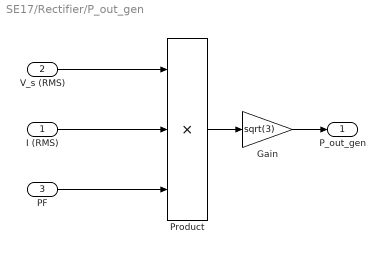
== system SE17/Rectifier/P_out_gen ==
  I (RMS) : Inport
  V_s (RMS) : Inport  Port=2
  PF : Inport  Port=3
  Gain : Gain  Gain=sqrt(3)
  Product : Product  Inputs=3
  P_out_gen : Outport  VectorParamsAs1DForOutWhenUnconnected=off
  wires:
  I (RMS)/1 -> Product/2
  PF/1 -> Product/3
  V_s (RMS)/1 -> Product/1
  Gain/1 -> P_out_gen/1
  Product/1 -> Gain/1

== system SE17/Rectifier/mVal ==
  V_s : Inport
  V_batt : Inport  Port=2
  Divide : Product  Inputs=*/
  Gain : Gain  Gain=sqrt(2)
  m : Outport  VectorParamsAs1DForOutWhenUnconnected=off
  wires:
  Divide/1 -> m/1
  V_s/1 -> Gain/1
  Gain/1 -> Divide/1
  V_batt/1 -> Divide/2

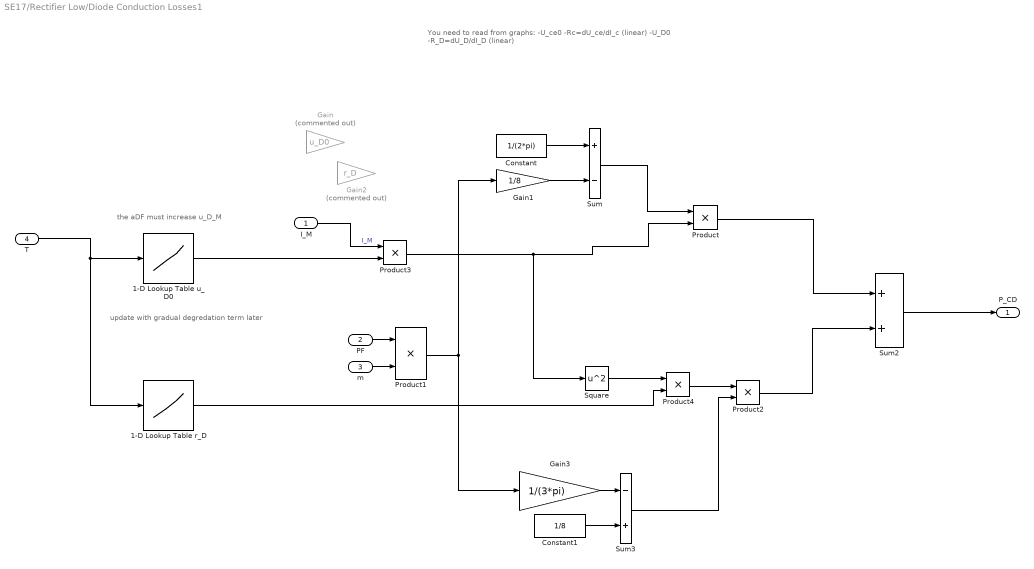
== system SE17/Rectifier Low/Diode Conduction Losses1 ==
  note: You need to read from graphs:
      |
      | -U_ce0
      | -Rc=dU_ce/dI_c (linear)
      | -U_D0
      | -R_D=dU_D/dI_D (linear)
  note: the aDF must increase u_D_M
  note: update with gradual degredation term later
  I_M : Inport
  PF : Inport  Port=2
  m : Inport  Port=3
  T : Inport  Port=4
  1-D Lookup Table r_D : Lookup_n-D  NumberOfTableDimensions=1  BreakpointsForDimension1=T_M  Table=R_D_M  InternalRulePriority=Speed  RndMeth=Simplest  InputSameDT=on
  1-D Lookup Table u_D0 : Lookup_n-D  NumberOfTableDimensions=1  BreakpointsForDimension1=T_M  Table=u_D_M  InternalRulePriority=Speed  RndMeth=Simplest  InputSameDT=on
  Constant : Constant  Value=1/(2*pi)
  Constant1 : Constant  Value=1/8
  Gain : Gain  Commented=on  Gain=u_D0
  Gain1 : Gain  Gain=1/8
  Gain2 : Gain  Commented=on  Gain=r_D
  Gain3 : Gain  Gain=1/(3*pi)
  Product{,1..4} (5 alike) : Product
  Square : Math  Operator=square  SignedPower=on  SaturateOnIntegerOverflow=on
  Sum : Sum  Inputs=+-
  Sum2 : Sum
  Sum3 : Sum  Inputs=-+
  P_CD : Outport  VectorParamsAs1DForOutWhenUnconnected=off
  wires:
  Product/1 -> Sum2/1
  Product2/1 -> Sum2/2
  Sum2/1 -> P_CD/1
  I_M/1 -> Product3/1  "I_M"
  Product3/1 -> Product/2, Square/1
  Constant/1 -> Sum/1
  PF/1 -> Product1/1
  m/1 -> Product1/2
  Gain1/1 -> Sum/2
  Product1/1 -> Gain3/1, Gain1/1
  Sum/1 -> Product/1
  Square/1 -> Product4/1
  Gain3/1 -> Sum3/1
  Product4/1 -> Product2/1
  Constant1/1 -> Sum3/2
  Sum3/1 -> Product2/2
  T/1 -> 1-D Lookup Table u_D0/1, 1-D Lookup Table r_D/1
  1-D Lookup Table u_D0/1 -> Product3/2
  1-D Lookup Table r_D/1 -> Product4/2

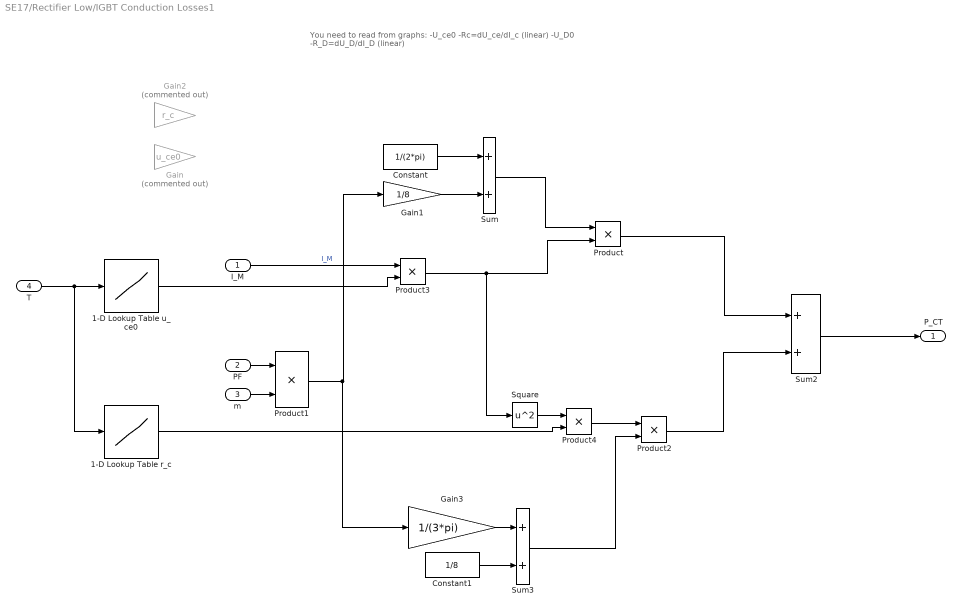
== system SE17/Rectifier Low/IGBT Conduction Losses1 ==
  note: You need to read from graphs:
      |
      | -U_ce0
      | -Rc=dU_ce/dI_c (linear)
      | -U_D0
      | -R_D=dU_D/dI_D (linear)
  I_M : Inport
  PF : Inport  Port=2
  m : Inport  Port=3
  T : Inport  Port=4
  1-D Lookup Table r_c : Lookup_n-D  NumberOfTableDimensions=1  BreakpointsForDimension1=T_M  Table=R_c_M  InternalRulePriority=Speed  RndMeth=Simplest  InputSameDT=on
  1-D Lookup Table u_ce0 : Lookup_n-D  NumberOfTableDimensions=1  BreakpointsForDimension1=T_M  Table=u_ce0_M  InternalRulePriority=Speed  RndMeth=Simplest  InputSameDT=on
  Constant : Constant  Value=1/(2*pi)
  Constant1 : Constant  Value=1/8
  Gain : Gain  Commented=on  Gain=u_ce0
  Gain1 : Gain  Gain=1/8
  Gain2 : Gain  Commented=on  Gain=r_c
  Gain3 : Gain  Gain=1/(3*pi)
  Product{,1..4} (5 alike) : Product
  Square : Math  Operator=square  SignedPower=on  SaturateOnIntegerOverflow=on
  Sum : Sum
  Sum2 : Sum
  Sum3 : Sum
  P_CT : Outport  VectorParamsAs1DForOutWhenUnconnected=off
  wires:
  Product/1 -> Sum2/1
  Product2/1 -> Sum2/2
  Sum2/1 -> P_CT/1
  I_M/1 -> Product3/1  "I_M"
  Product3/1 -> Product/2, Square/1
  Constant/1 -> Sum/1
  PF/1 -> Product1/1
  m/1 -> Product1/2
  Gain1/1 -> Sum/2
  Product1/1 -> Gain3/1, Gain1/1
  Sum/1 -> Product/1
  Square/1 -> Product4/1
  Gain3/1 -> Sum3/1
  Product4/1 -> Product2/1
  Constant1/1 -> Sum3/2
  Sum3/1 -> Product2/2
  T/1 -> 1-D Lookup Table u_ce0/1, 1-D Lookup Table r_c/1
  1-D Lookup Table u_ce0/1 -> Product3/2
  1-D Lookup Table r_c/1 -> Product4/2

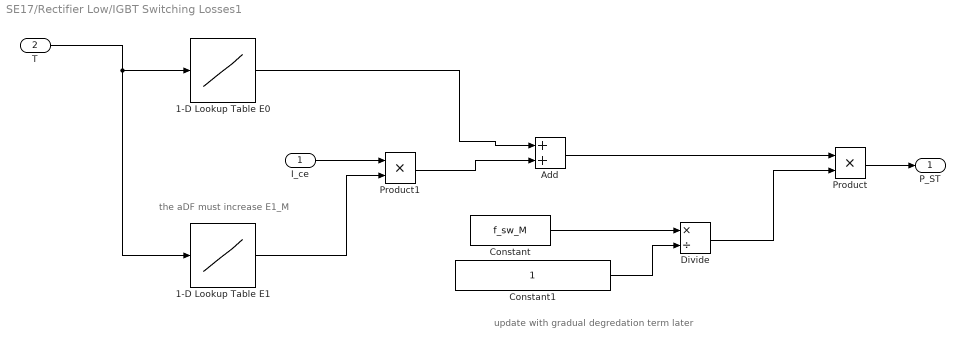
== system SE17/Rectifier Low/IGBT Switching Losses1 ==
  note: update with gradual degredation term later
  note: the aDF must increase E1_M
  I_ce : Inport
  T : Inport  Port=2
  1-D Lookup Table E0 : Lookup_n-D  NumberOfTableDimensions=1  BreakpointsForDimension1=T_M  Table=E0_M  InternalRulePriority=Speed  RndMeth=Simplest  InputSameDT=on
  1-D Lookup Table E1 : Lookup_n-D  NumberOfTableDimensions=1  BreakpointsForDimension1=T_M  Table=E1_M  InternalRulePriority=Speed  RndMeth=Simplest  InputSameDT=on
  Add : Sum
  Constant : Constant  Value=f_sw_M
  Constant1 : Constant
  Divide : Product  Inputs=*/
  Product : Product
  Product1 : Product
  P_ST : Outport  VectorParamsAs1DForOutWhenUnconnected=off
  wires:
  Constant1/1 -> Divide/2
  Divide/1 -> Product/2
  Constant/1 -> Divide/1
  1-D Lookup Table E1/1 -> Product1/2
  T/1 -> 1-D Lookup Table E1/1, 1-D Lookup Table E0/1
  Product1/1 -> Add/2
  1-D Lookup Table E0/1 -> Add/1
  I_ce/1 -> Product1/1
  Add/1 -> Product/1
  Product/1 -> P_ST/1
